simulink model "Copy_of_DCMotor"  (R2017a)
settings: Solver=FixedStepAuto  StartTime=0.0  StopTime=3  FixedStep=0.01  RelTol=1e-3
undefined symbols (not defined in the file or in its folder): J, K, L, R
settings Model: Creator=sansh  LastModifiedBy=nikhil

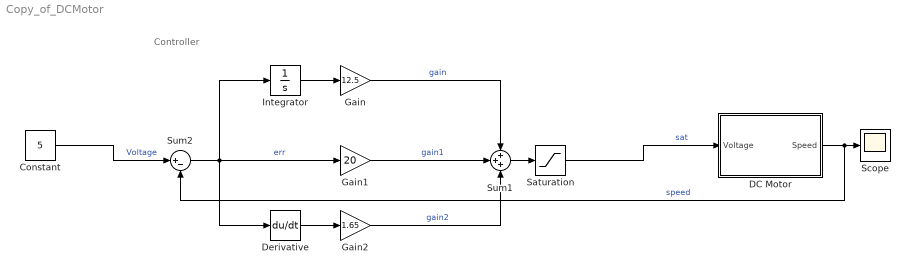
== system Copy_of_DCMotor ==
  note: Controller
  Constant : Constant  Value=5
  DC Motor : Subsystem
  Derivative : Derivative
  Gain : Gain  Gain=12.5
  Gain1 : Gain  Gain=20
  Gain2 : Gain  Gain=1.65
  Integrator : Integrator
  Saturation : Saturate  UpperLimit=15  LowerLimit=-15
  Scope : Scope
  Sum1 : Sum  Inputs=+++
  Sum2 : Sum  Inputs=|+-
  wires:
  Constant/1 -> Sum2/1  "Voltage"
  DC Motor/1(Speed) -> Scope/1, Sum2/2  "speed"
  Saturation/1 -> DC Motor/1(Voltage)  "sat"
  Gain/1 -> Sum1/1  "gain"
  Gain2/1 -> Sum1/3  "gain2"
  Integrator/1 -> Gain/1
  Sum2/1 -> Derivative/1, Gain1/1, Integrator/1  "err"
  Derivative/1 -> Gain2/1
  Sum1/1 -> Saturation/1
  Gain1/1 -> Sum1/2  "gain1"

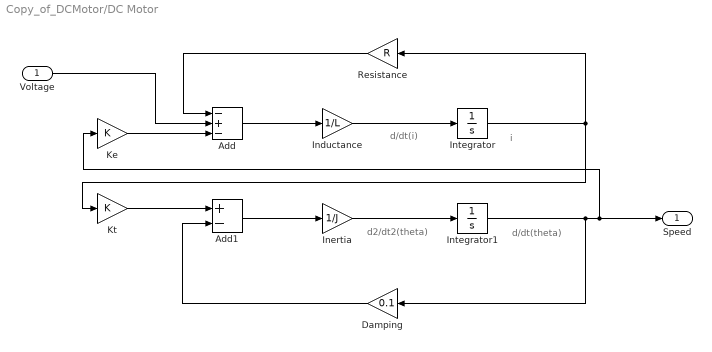
== system Copy_of_DCMotor/DC Motor ==
  note: i
  note: d/dt(i)
  note: d/dt(theta)
  note: d2/dt2(theta)
  Voltage : Inport
  Add : Sum  Inputs=-+-
  Add1 : Sum  Inputs=+-
  Damping : Gain  Gain=0.1
  Inductance : Gain  Gain=1/L
  Inertia : Gain  Gain=1/J
  Integrator : Integrator
  Integrator1 : Integrator
  Ke : Gain  Gain=K
  Kt : Gain  Gain=K
  Resistance : Gain  Gain=R
  Speed : Outport
  wires:
  Inductance/1 -> Integrator/1
  Integrator1/1 -> Damping/1, Speed/1, Ke/1
  Inertia/1 -> Integrator1/1
  Integrator/1 -> Resistance/1, Kt/1
  Kt/1 -> Add1/1
  Voltage/1 -> Add/2
  Resistance/1 -> Add/1
  Damping/1 -> Add1/2
  Ke/1 -> Add/3
  Add/1 -> Inductance/1
  Add1/1 -> Inertia/1
